simulink model "Satellite_model_simulink_1_1"  (R2025b)
settings: Solver=VariableStepAuto  StartTime=0.0  StopTime=10.0  RelTol=1e-3
undefined symbols (not defined in the file or in its folder): alpha, Js, omega, xi
settings Model: Creator=flori  LastModifiedBy=flori

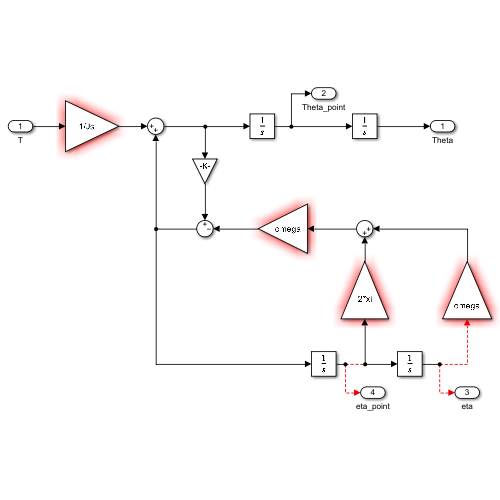
[thumbnail: Simulink's stored preview of the top-level diagram]
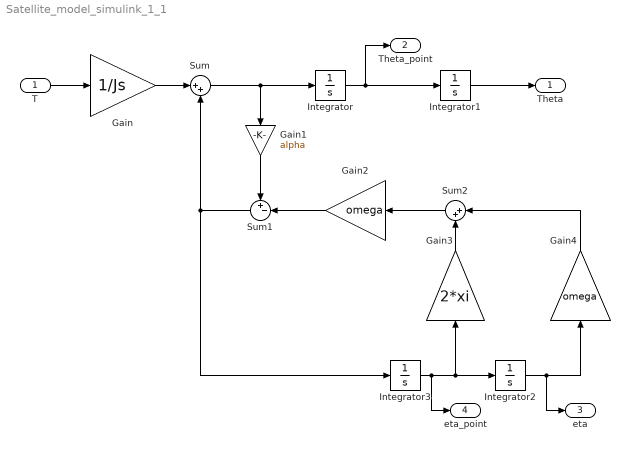
== system Satellite_model_simulink_1_1 ==
  T : Inport
  Gain : Gain  Gain=1/Js
  Gain1 : Gain  Gain=alpha
  Gain2 : Gain  Gain=omega
  Gain3 : Gain  Gain=2*xi
  Gain4 : Gain  Gain=omega
  Integrator{,1..3} (4 alike) : Integrator
  Sum : Sum  Inputs=|++
  Sum1 : Sum  Inputs=+-|
  Sum2 : Sum  Inputs=|++
  Theta : Outport
  Theta_point : Outport  Port=2
  eta : Outport  Port=3
  eta_point : Outport  Port=4
  wires:
  T/1 -> Gain/1
  Gain/1 -> Sum/1
  Integrator/1 -> Integrator1/1, Theta_point/1
  Integrator1/1 -> Theta/1
  Gain4/1 -> Sum2/1
  Gain3/1 -> Sum2/2
  Integrator2/1 -> eta/1, Gain4/1
  Gain2/1 -> Sum1/2
  Sum2/1 -> Gain2/1
  Gain1/1 -> Sum1/1
  Sum/1 -> Gain1/1, Integrator/1
  Integrator3/1 -> eta_point/1, Integrator2/1, Gain3/1
  Sum1/1 -> Integrator3/1, Sum/2
